simulink model "test"  (R2019b)
settings: Solver=VariableStepAuto  StartTime=0.0  StopTime=10.0  RelTol=1e-3
settings Model: Creator=15656  LastModifiedBy=15656

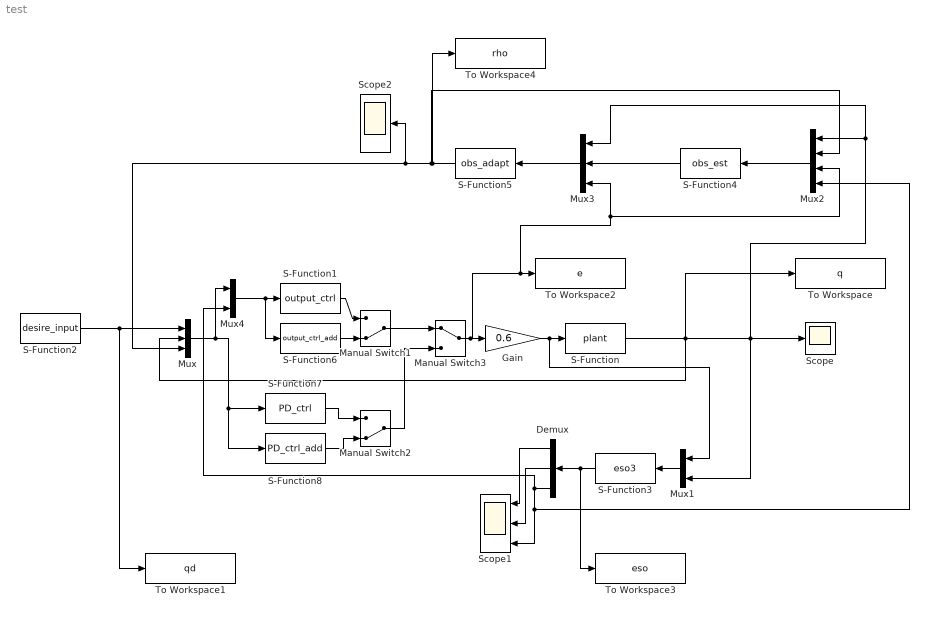
== system test ==
  Demux : Demux  Outputs=3
  Gain : Gain  Gain=0.6
  Manual Switch1 : ManualSwitch  CurrentSetting=0
  Manual Switch2 : ManualSwitch  CurrentSetting=0
  Manual Switch3 : ManualSwitch
  Mux : Mux  Inputs=3
  Mux1 : Mux  Inputs=2
  Mux2 : Mux
  Mux3 : Mux  Inputs=3
  Mux4 : Mux  Inputs=2
  S-Function : S-Function  FunctionName=plant  SFunctionDeploymentMode=off  EnableBusSupport=off
  S-Function1 : S-Function  FunctionName=output_ctrl  SFunctionDeploymentMode=off  EnableBusSupport=off
  S-Function2 : S-Function  FunctionName=desire_input  SFunctionDeploymentMode=off  EnableBusSupport=off
  S-Function3 : S-Function  FunctionName=eso3  SFunctionDeploymentMode=off  EnableBusSupport=off
  S-Function4 : S-Function  FunctionName=obs_est  SFunctionDeploymentMode=off  EnableBusSupport=off
  S-Function5 : S-Function  FunctionName=obs_adapt  SFunctionDeploymentMode=off  EnableBusSupport=off
  S-Function6 : S-Function  FunctionName=output_ctrl_add  SFunctionDeploymentMode=off  EnableBusSupport=off
  S-Function7 : S-Function  FunctionName=PD_ctrl  SFunctionDeploymentMode=off  EnableBusSupport=off
  S-Function8 : S-Function  FunctionName=PD_ctrl_add  SFunctionDeploymentMode=off  EnableBusSupport=off
  Scope : Scope
  Scope1 : Scope  NumInputPorts=3
  Scope2 : Scope
  To Workspace : ToWorkspace  VariableName=q  SaveFormat=Timeseries  SampleTime=-1
  To Workspace1 : ToWorkspace  VariableName=qd  SaveFormat=Timeseries  SampleTime=-1
  To Workspace2 : ToWorkspace  VariableName=e  SaveFormat=Timeseries  SampleTime=-1
  To Workspace3 : ToWorkspace  VariableName=eso  SaveFormat=Timeseries  SampleTime=-1
  To Workspace4 : ToWorkspace  VariableName=rho  SaveFormat=Timeseries  SampleTime=-1
  wires:
  Mux/1 -> Mux4/1, S-Function7/1, S-Function8/1
  S-Function2/1 -> To Workspace1/1, Mux/1
  S-Function/1 -> To Workspace/1, Mux/2, Mux2/1, Mux3/1, Mux1/2, Scope/1
  S-Function1/1 -> Manual Switch1/1
  Gain/1 -> Mux1/1, S-Function/1
  Mux1/1 -> S-Function3/1
  S-Function3/1 -> To Workspace3/1, Demux/1
  Demux/1 -> Scope1/1
  Demux/2 -> Scope1/2
  Demux/3 -> Mux2/4, Scope1/3, Mux4/2
  Mux3/1 -> S-Function5/1
  S-Function4/1 -> Mux3/2
  Mux2/1 -> S-Function4/1
  S-Function5/1 -> To Workspace4/1, Mux/3, Scope2/1, Mux2/2
  S-Function6/1 -> Manual Switch1/2
  S-Function7/1 -> Manual Switch2/1
  S-Function8/1 -> Manual Switch2/2
  Manual Switch1/1 -> Manual Switch3/1
  Manual Switch2/1 -> Manual Switch3/2
  Manual Switch3/1 -> Mux3/3, Mux2/3, To Workspace2/1, Gain/1
  Mux4/1 -> S-Function6/1, S-Function1/1
